simulink model "FuzzyPID"  (R2024a)
settings: Solver=VariableStepAuto  StartTime=0.0  StopTime=1000  RelTol=1e-3
libraries: fuzblock x2, slpidlib x1
settings Model: Creator=Korisnik  LastModifiedBy=Korisnik

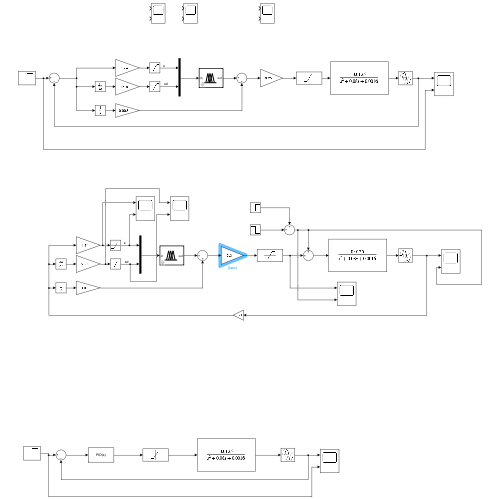
[thumbnail: Simulink's stored preview of the top-level diagram]
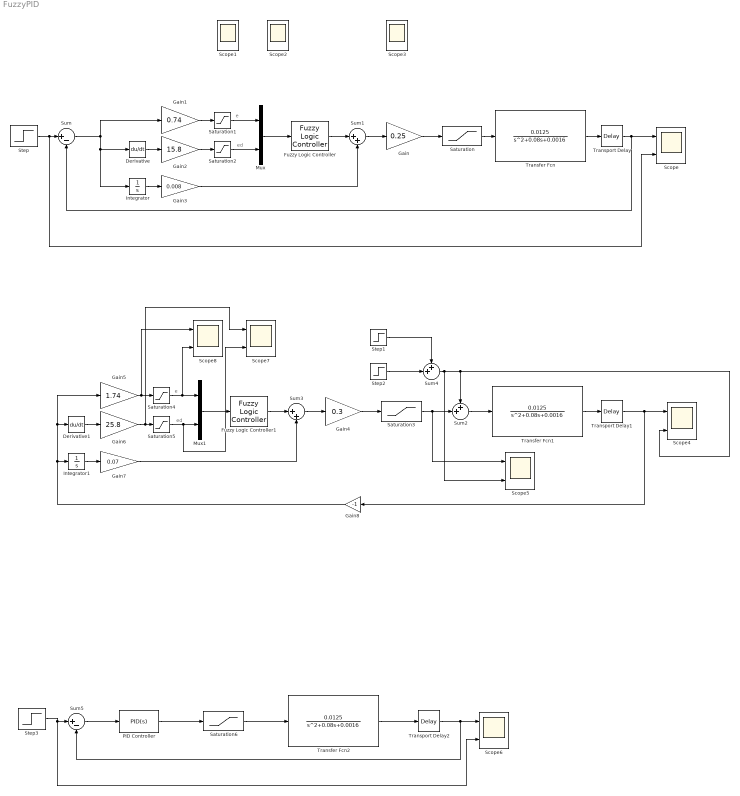
== system FuzzyPID ==
  note: ed
  note: e
  note: e
  note: ed
  Derivative : Derivative
  Derivative1 : Derivative
  Fuzzy Logic Controller : fuzblock/Fuzzy Logic  Controller  FIS='sugenoFIS.fis'  OutputSampleNumber=101  DataType=double  FuzzifiedInputs=off  RuleFiringStrengths=off  RuleOutputs=off  AggregatedOutputs=off  SimulateUsing=Interpreted execution  OutOfRangeInputValueMessage=warning  NoRuleFiredMessage=warning  EmptyOutputFuzzySetMessage=warning
  Fuzzy Logic Controller1 : fuzblock/Fuzzy Logic  Controller  FIS='sugenoFIS.fis'  OutputSampleNumber=101  DataType=double  FuzzifiedInputs=off  RuleFiringStrengths=off  RuleOutputs=off  AggregatedOutputs=off  SimulateUsing=Interpreted execution  OutOfRangeInputValueMessage=warning  NoRuleFiredMessage=warning  EmptyOutputFuzzySetMessage=warning
  Gain : Gain  Gain=0.25
  Gain1 : Gain  Gain=0.74
  Gain2 : Gain  Gain=15.8
  Gain3 : Gain  Gain=0.008
  Gain4 : Gain  Gain=0.3
  Gain5 : Gain  Gain=1.74
  Gain6 : Gain  Gain=25.8
  Gain7 : Gain  Gain=0.07
  Gain8 : Gain  Gain=-1
  Integrator : Integrator
  Integrator1 : Integrator
  Mux : Mux  Inputs=2
  Mux1 : Mux  Inputs=2
  PID Controller : slpidlib/PID Controller  Controller=PID  Form=Parallel  TimeDomain=Continuous-time  UseExternalTs=off  SampleTime=-1  IntegratorMethod=Forward Euler  FilterMethod=Forward Euler  ControllerParametersSource=internal  P=0.436  I=0.012  UseKiTs=off  D=3.95  UseExternalDerivativeSource=off  N=100  UseFilter=on  TunerSelectOption=Transfer Function Based (PID Tuner App)  InitialConditionSource=internal  InitialConditionForIntegrator=0  InitialConditionForFilter=0  DifferentiatorICPrevScaledInput=0  ExternalReset=none  TrackingMode=off  Kt=1  LimitOutput=off  SatLimitsSource=internal  UpperSaturationLimit=inf  LowerSaturationLimit=-inf  LinearizeAsGain=on  AntiWindupMode=none  Kb=1  LimitIntegrator=off  UpperIntegratorSaturationLimit=inf  LowerIntegratorSaturationLimit=-inf  POutMin=[]  POutMax=[]  IOutMin=[]  IOutMax=[]  DOutMin=[]  DOutMax=[]  NOutMin=[]  NOutMax=[]  SumOutMin=[]  SumOutMax=[]  SaturationOutMin=[]  SaturationOutMax=[]  PParamMin=[]  PParamMax=[]  IParamMin=[]  IParamMax=[]  DParamMin=[]  DParamMax=[]  NParamMin=[]  NParamMax=[]  KbParamMin=[]  KbParamMax=[]  KtParamMin=[]  KtParamMax=[]  KbOutMin=[]  KbOutMax=[]  KtOutMin=[]  KtOutMax=[]  IntegratorOutMin=[]  IntegratorOutMax=[]  FilterOutMin=[]  FilterOutMax=[]  SumI1OutMin=[]  SumI1OutMax=[]  SumI2OutMin=[]  SumI2OutMax=[]  SumI3OutMin=[]  SumI3OutMax=[]  SumI4OutMin=[]  SumI4OutMax=[]  SumDOutMin=[]  SumDOutMax=[]  DifferentiatorOutMin=[]  DifferentiatorOutMax=[]  FilterDiffOutCoefMin=[]  FilterDiffOutCoefMax=[]  ReciprocalOutMin=[]  ReciprocalOutMax=[]  SumDenOutMin=[]  SumDenOutMax=[]  SumNumOutMin=[]  SumNumOutMax=[]  DivideOutMin=[]  DivideOutMax=[]  UdiffTsProdOutMin=[]  UdiffTsProdOutMax=[]  NTsProdOutMin=[]  NTsProdOutMax=[]  UintegralTsProdOutMin=[]  UintegralTsProdOutMax=[]  UngainTsProdOutMin=[]  UngainTsProdOutMax=[]  ClampingZeroOutDataTypeStr=Inherit: Inherit via back propagation  ClampingZeroOutMin=[]  ClampingZeroOutMax=[]  FilterDenConstantOutDataTypeStr=Inherit: Inherit via back propagation  FilterDenConstantOutMin=[]  FilterDenConstantOutMax=[]  PCopyOutDataTypeStr=Inherit: Inherit via back propagation  PCopyOutMin=[]  PCopyOutMax=[]  NCopyOutDataTypeStr=Inherit: Inherit via back propagation  NCopyOutMin=[]  NCopyOutMax=[]  IntegratorContinuousStateAttributes=''  IntegratorStateMustResolveToSignalObject=off  IntegratorRTWStateStorageClass=Auto  FilterContinuousStateAttributes=''  FilterStateMustResolveToSignalObject=off  FilterRTWStateStorageClass=Auto  ParallelPVariant=InternalParameters  IdealPVariant=Disabled  IVariant=InternalParameters  DVariant=InternalParameters  IntegratorVariant=Continuous  SatVariant=Disabled  AWVariant=Passthrough  PCopyVariant=Disabled  TRVariant=Disabled  FdbkBlocksVariant=Forward  IdealPFdbkVariant=Disabled  SatFdbkVariant=Disabled  DerivativeFilterVariant=ContFilter  NVariant=InternalParameters  NCopyVariant=Disabled  FilterICVariant=InternalICsFilter  IntegratorICVariant=InternalICs  ExternalResetVariant=Disabled  TRSumVariant=Passthrough  SumFdbkVariant=Disabled  SumVariant=Sum_PID  TsampFilterVariant=InternalTs  TsampNgainVariant=Passthrough  TsampIntegralVariant=Disabled_SignalSpec  ExternalSaturationOutDataTypeStr=Inherit: Same as second input  DerivativeSourceVariant=ErrorSignal
  Saturation : Saturate
  Saturation{1..2,4..5} (4 alike) : Saturate  UpperLimit=1  LowerLimit=-1
  Saturation3 : Saturate
  Saturation6 : Saturate
  Scope{,1..8} (9 alike) : Scope  NumInputPorts=2
  Step : Step  Time=300  Before=-2  After=2  SampleTime=0
  Step1 : Step  Time=100  After=0.25  SampleTime=0
  Step2 : Step  Time=600  After=-0.5  SampleTime=0
  Step3 : Step  Time=300  Before=-2  After=2  SampleTime=0
  Sum : Sum  Inputs=|+-
  Sum1 : Sum  Inputs=|++
  Sum2 : Sum  Inputs=++|
  Sum3 : Sum  Inputs=|++
  Sum4 : Sum  Inputs=++|
  Sum5 : Sum  Inputs=|+-
  Transfer Fcn : TransferFcn  Numerator=[0.0125]  Denominator=[1 0.08 0.0016]
  Transfer Fcn1 : TransferFcn  Numerator=[0.0125]  Denominator=[1 0.08 0.0016]
  Transfer Fcn2 : TransferFcn  Numerator=[0.0125]  Denominator=[1 0.08 0.0016]
  Transport Delay : TransportDelay  DelayTime=10
  Transport Delay1 : TransportDelay  DelayTime=10
  Transport Delay2 : TransportDelay  DelayTime=10
  wires:
  Step/1 -> Scope/2, Sum/1
  Transfer Fcn/1 -> Transport Delay/1
  Saturation/1 -> Transfer Fcn/1
  Fuzzy Logic Controller/1 -> Sum1/1
  Gain/1 -> Saturation/1
  Sum1/1 -> Gain/1
  Gain1/1 -> Saturation1/1
  Gain2/1 -> Saturation2/1
  Derivative/1 -> Gain2/1
  Sum/1 -> Integrator/1, Derivative/1, Gain1/1
  Integrator/1 -> Gain3/1
  Gain3/1 -> Sum1/2
  Saturation1/1 -> Mux/1
  Saturation2/1 -> Mux/2
  Mux/1 -> Fuzzy Logic Controller/1
  Mux1/1 -> Fuzzy Logic Controller1/1
  Saturation4/1 -> Scope8/2, Mux1/1
  Derivative1/1 -> Gain6/1
  Gain7/1 -> Sum3/2
  Gain5/1 -> Scope8/1, Saturation4/1
  Gain6/1 -> Scope7/1, Saturation5/1
  Integrator1/1 -> Gain7/1
  Fuzzy Logic Controller1/1 -> Sum3/1
  Saturation5/1 -> Scope7/2, Mux1/2
  Gain4/1 -> Saturation3/1
  Sum3/1 -> Gain4/1
  Transfer Fcn1/1 -> Transport Delay1/1
  Sum2/1 -> Transfer Fcn1/1
  Step1/1 -> Sum4/1
  Step2/1 -> Sum4/2
  Saturation3/1 -> Scope5/1, Sum2/2
  Sum4/1 -> Scope5/2, Sum2/1, Scope4/2
  Transport Delay1/1 -> Gain8/1, Scope4/1
  Gain8/1 -> Gain5/1, Derivative1/1, Integrator1/1
  Transport Delay/1 -> Sum/2, Scope/1
  Transport Delay2/1 -> Scope6/1, Sum5/2
  Saturation6/1 -> Transfer Fcn2/1
  Step3/1 -> Scope6/2, Sum5/1
  Transfer Fcn2/1 -> Transport Delay2/1
  Sum5/1 -> PID Controller/1
  PID Controller/1 -> Saturation6/1
